simulink model "Case2_AlgebraicLoop"  (R2021a)
settings: Solver=ode2  StartTime=0.0  StopTime=0.05  FixedStep=1000e-6  RelTol=1e-3
settings Model: Creator=s.ebrahimi  LastModifiedBy=s.ebrahimi
settings DebuggingCC: AlgebraicLoopMsg=none  UnconnectedInputMsg=none  UnconnectedOutputMsg=none  UnconnectedLineMsg=none
settings ModelReferenceCC: EnableRefExpFcnMdlSchedulingChecks=off
settings RTWCC: Description=Generic Real-Time Target  GPUComputeCapability=5.0  DLArmComputeVersion=20.02.1

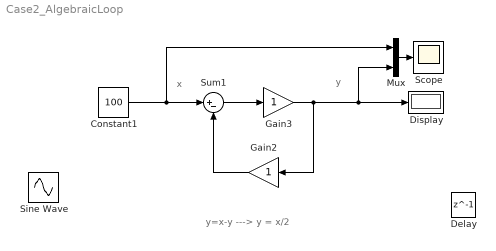
== system Case2_AlgebraicLoop ==
  note: y=x-y ---> y = x/2
  note: y
  note: x
  Constant1 : Constant  Value=100
  Delay : Delay  DelayLength=1  InitialCondition=0
  Display : Display
  Gain2 : Gain
  Gain3 : Gain
  Mux : Mux  Inputs=2
  Scope : Scope
  Sine Wave : Sin  Amplitude=100  Frequency=600  SampleTime=0
  Sum1 : Sum  Inputs=|+-
  wires:
  Constant1/1 -> Mux/1, Sum1/1
  Gain2/1 -> Sum1/2
  Sum1/1 -> Gain3/1
  Mux/1 -> Scope/1
  Gain3/1 -> Gain2/1, Display/1, Mux/2
